simulink model "BME331Lab3_Update"  (R2023a)
settings: Solver=ode5  StartTime=0.0  StopTime=120  FixedStep=1/960  RelTol=1e-3
settings Model: SimulationMode=rapid-accelerator  Creator=ihass  LastModifiedBy=ihass

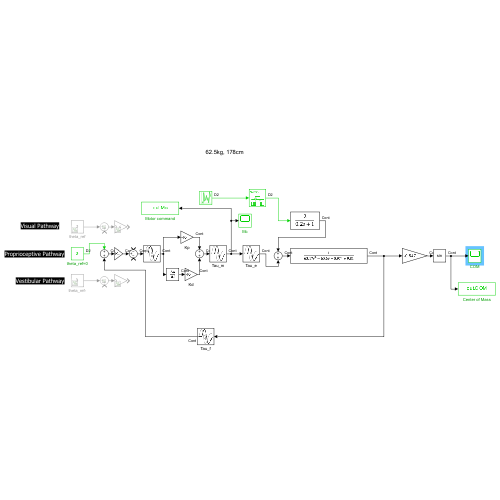
[thumbnail: Simulink's stored preview of the top-level diagram]
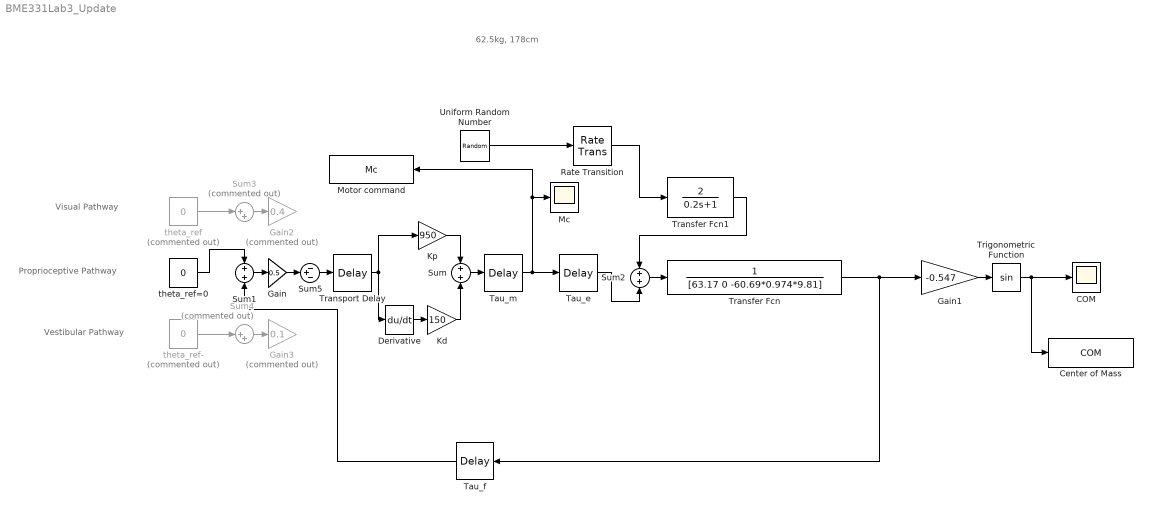
== system BME331Lab3_Update ==
  note: Proprioceptive Pathway
  note: 62.5kg, 178cm
  note: Visual Pathway
  note: Vestibular Pathway
  COM : Scope
  Center of Mass : ToWorkspace  VariableName=COM  SampleTime=0.1
  Derivative : Derivative
  Gain : Gain  Gain=0.5
  Gain1 : Gain  Gain=-0.547
  Gain2 : Gain  Commented=on  Gain=0.4
  Gain3 : Gain  Commented=on  Gain=0.1
  Kd : Gain  Gain=150
  Kp : Gain  Gain=950
  Mc : Scope
  Motor command : ToWorkspace  VariableName=Mc  SampleTime=0.1
  Rate Transition : RateTransition  OutPortSampleTime=0.1
  Sum : Sum  Inputs=+|+
  Sum1 : Sum  Inputs=+|+
  Sum2 : Sum  Inputs=+|+
  Sum3 : Sum  Commented=on  Inputs=|++
  Sum4 : Sum  Commented=on  Inputs=|++
  Sum5 : Sum  Inputs=-+-
  Tau_e : TransportDelay  DelayTime=0.01
  Tau_f : TransportDelay  DelayTime=0.04
  Tau_m : TransportDelay  DelayTime=0.05
  Transfer Fcn : TransferFcn  Denominator=[63.17 0 -60.69*0.974*9.81]
  Transfer Fcn1 : TransferFcn  Numerator=[2]  Denominator=[0.2 1]
  Transport Delay : TransportDelay
  Trigonometric Function : Trigonometry
  Uniform Random Number : UniformRandomNumber  Minimum=-4  Maximum=4  SampleTime=0.1
  theta_ref : Constant  Commented=on  Value=0  SampleTime=0.1
  theta_ref- : Constant  Commented=on  Value=0  SampleTime=0.1
  theta_ref=0 : Constant  Value=0  SampleTime=0.1
  wires:
  Kd/1 -> Sum/2
  Kp/1 -> Sum/1
  Derivative/1 -> Kd/1
  Transfer Fcn/1 -> Gain1/1, Tau_f/1
  Gain1/1 -> Trigonometric Function/1
  Sum/1 -> Tau_m/1
  Uniform Random Number/1 -> Rate Transition/1
  Rate Transition/1 -> Transfer Fcn1/1
  Tau_e/1 -> Sum2/2
  Transfer Fcn1/1 -> Sum2/1
  Sum2/1 -> Transfer Fcn/1
  Tau_m/1 -> Mc/1, Motor command/1, Tau_e/1
  Trigonometric Function/1 -> Center of Mass/1, COM/1
  Transport Delay/1 -> Kp/1, Derivative/1
  Sum1/1 -> Gain/1
  theta_ref/1 -> Sum3/1
  theta_ref=0/1 -> Sum1/1
  Sum3/1 -> Gain2/1
  theta_ref-/1 -> Sum4/1
  Sum5/1 -> Transport Delay/1
  Sum4/1 -> Gain3/1
  Tau_f/1 -> Sum1/2
  Gain/1 -> Sum5/2
